simulink model "geared_motor_load_fixed"  (R2023b)
settings: Solver=VariableStepAuto  StartTime=0.0  StopTime=1  RelTol=1e-3
values from neighbouring files (symbols this model uses):
  angle_ref = Angle_reference_values(i)    [homework_three.m]
  B_load = 0    [homework_three.m]
  Beq = Jeq / 0.00376    (= 0.00264630474582)    [homework_three.m]
  gain = gear_ratio    (= 0.0123456790123)    [homework_three.m]
  gear_alpha = 0.72    [homework_three.m]
  gear_ratio = 1/81    (= 0.0123456790123)    [homework_three.m]
  J_load = 0    [homework_three.m]
  Jeq = Jm + (1 / gear_alpha) * gear_ratio * gear_ratio * Jg    (= 9.9501058443e-06)    [homework_three.m]
  Ka_c = 1 / Kp_c    (= 2.41883946985)    [homework_three.m]
  Ka_v = 1/Kp_v    (= 289.1342348)    [homework_three.m]
  Kd_p = wcp/wcv    (= 0.1)    [homework_three.m]
  Ke = 0.0683    [homework_three.m]
  Ki_c = Ra * wcc    (= 1105.808)    [homework_three.m]
  Ki_v = (Beq+(B_load*0.00021))*wcv*81/Kt    (= 197.183799438)    [homework_three.m]
  Kp_c = La * wcc    (= 0.4134214)    [homework_three.m]
  Kp_p = wcp    (= 6.283)    [homework_three.m]
  Kp_v = (Jeq+(J_load*0.00021))*wcv*81*Kt    (= 0.00345860116044)    [homework_three.m]
  Kt = 0.0683    [homework_three.m]
  La = 0.000658    [homework_three.m]
  Ra = 1.76    [homework_three.m]
settings Model: Creator=junseo  LastModifiedBy=minjs
settings SolverCC: ZeroCrossAlgorithm=Adaptive
settings OptimizationCC: ReuseModelBlockBuffer=off
settings DebuggingCC: IgnoredZcDiagnostic=none

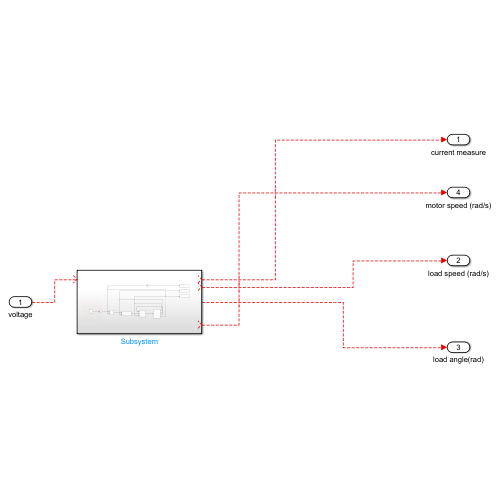
[thumbnail: Simulink's stored preview of the top-level diagram]
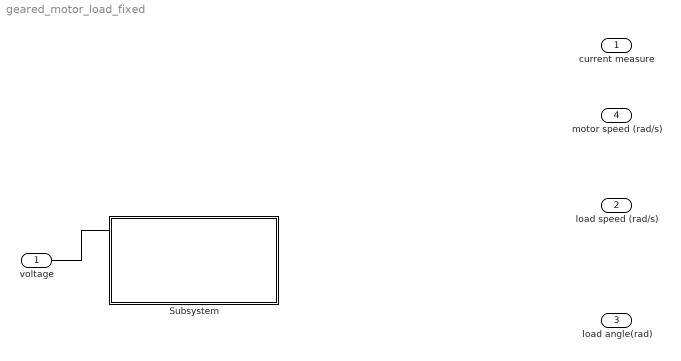
== system geared_motor_load_fixed ==
  voltage : Inport
  Subsystem : Subsystem
  current measure : Outport
  load speed (rad/s) : Outport  Port=2
  load angle(rad) : Outport  Port=3
  motor speed (rad/s) : Outport  Port=4
  wires:
  voltage/1 -> ?
  ? -> current measure/1
  ? -> load speed (rad/s)/1
  ? -> load angle(rad)/1
  ? -> motor speed (rad/s)/1

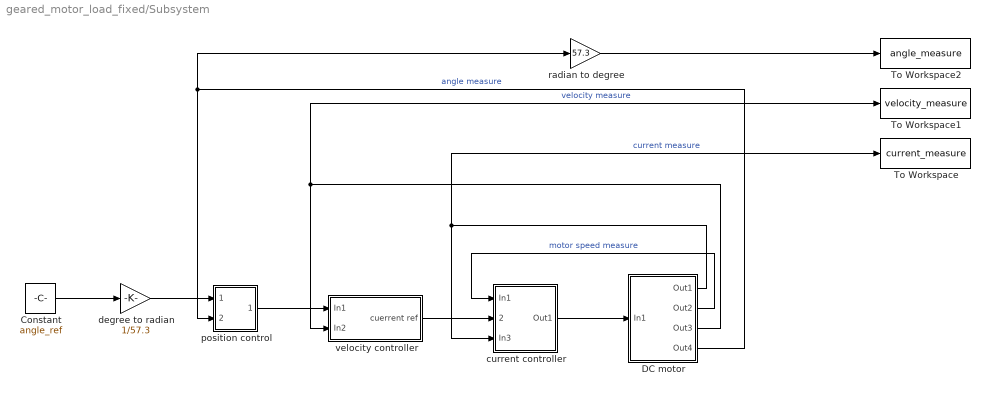
== system geared_motor_load_fixed/Subsystem ==
  Constant : Constant  Value=angle_ref
  DC motor : Subsystem
  To Workspace : ToWorkspace  VariableName=current_measure  SaveFormat=Timeseries  SampleTime=-1
  To Workspace1 : ToWorkspace  VariableName=velocity_measure  SaveFormat=Timeseries  SampleTime=-1
  To Workspace2 : ToWorkspace  VariableName=angle_measure  SaveFormat=Timeseries  SampleTime=-1
  current controller : Subsystem
  degree to radian : Gain  Gain=1/57.3
  position control : Subsystem
  radian to degree : Gain  Gain=57.3
  velocity controller : Subsystem
  wires:
  current controller/1(Out1) -> DC motor/1(In1)
  DC motor/2(Out2) -> current controller/1(In1)  "motor speed measure"
  DC motor/1(Out1) -> To Workspace/1, current controller/3(In3)  "current measure"
  position control/1(Out1) -> velocity controller/1(In1)
  DC motor/3(Out3) -> To Workspace1/1, velocity controller/2(In2)  "velocity measure"
  velocity controller/1(cuerrent ref) -> current controller/2(cuerrent ref)
  Constant/1 -> degree to radian/1
  DC motor/4(Out4) -> radian to degree/1, position control/2(In2)  "angle measure"
  radian to degree/1 -> To Workspace2/1
  degree to radian/1 -> position control/1(In1)

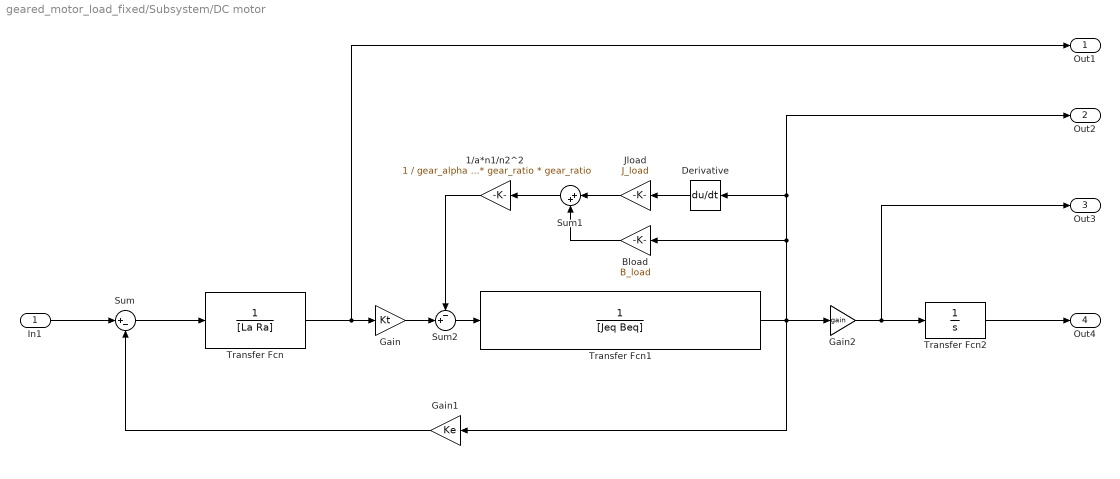
== system geared_motor_load_fixed/Subsystem/DC motor ==
  In1 : Inport
  1/a*n1/n2^2 : Gain  Gain=1 / gear_alpha * gear_ratio * gear_ratio
  Bload : Gain  Gain=B_load
  Derivative : Derivative
  Gain : Gain  Gain=Kt
  Gain1 : Gain  Gain=Ke
  Gain2 : Gain  Gain=gain
  Jload : Gain  Gain=J_load
  Sum : Sum  Inputs=|+-
  Sum1 : Sum  Inputs=|++
  Sum2 : Sum  Inputs=-+|
  Transfer Fcn : TransferFcn  Denominator=[La Ra]
  Transfer Fcn1 : TransferFcn  Denominator=[Jeq Beq]
  Transfer Fcn2 : TransferFcn  Denominator=[1 0]
  Out1 : Outport
  Out2 : Outport  Port=2
  Out3 : Outport  Port=3
  Out4 : Outport  Port=4
  wires:
  Jload/1 -> Sum1/1
  Gain1/1 -> Sum/2
  Bload/1 -> Sum1/2
  Sum2/1 -> Transfer Fcn1/1
  Gain2/1 -> Out3/1, Transfer Fcn2/1
  Derivative/1 -> Jload/1
  Transfer Fcn1/1 -> Gain1/1, Gain2/1, Bload/1, Out2/1, Derivative/1
  Transfer Fcn/1 -> Out1/1, Gain/1
  Sum1/1 -> 1/a*n1/n2^2/1
  1/a*n1/n2^2/1 -> Sum2/1
  Gain/1 -> Sum2/2
  Sum/1 -> Transfer Fcn/1
  Transfer Fcn2/1 -> Out4/1
  In1/1 -> Sum/1

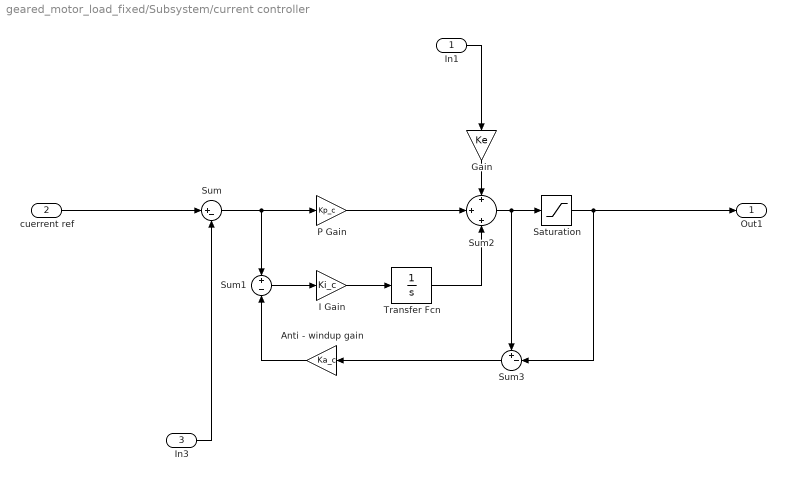
== system geared_motor_load_fixed/Subsystem/current controller ==
  In1 : Inport
  cuerrent ref : Inport  Port=2
  In3 : Inport  Port=3
  Anti - windup gain : Gain  Gain=Ka_c
  Gain : Gain  Gain=Ke
  I Gain : Gain  Gain=Ki_c
  P Gain : Gain  Gain=Kp_c
  Saturation : Saturate  UpperLimit=48  LowerLimit=-48
  Sum : Sum  Inputs=|+-
  Sum1 : Sum  Inputs=+|-
  Sum2 : Sum  Inputs=+|+|+
  Sum3 : Sum  Inputs=+-|
  Transfer Fcn : TransferFcn  Denominator=[1 0]
  Out1 : Outport
  wires:
  cuerrent ref/1 -> Sum/1
  I Gain/1 -> Transfer Fcn/1
  Transfer Fcn/1 -> Sum2/3
  Sum1/1 -> I Gain/1
  Sum/1 -> Sum1/1, P Gain/1
  Gain/1 -> Sum2/1
  P Gain/1 -> Sum2/2
  Saturation/1 -> Out1/1, Sum3/2
  In1/1 -> Gain/1
  Sum2/1 -> Saturation/1, Sum3/1
  Sum3/1 -> Anti - windup gain/1
  Anti - windup gain/1 -> Sum1/2
  In3/1 -> Sum/2

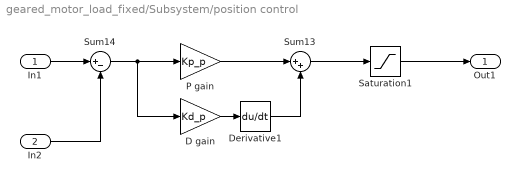
== system geared_motor_load_fixed/Subsystem/position control ==
  In1 : Inport
  In2 : Inport  Port=2
  D gain : Gain  Gain=Kd_p
  Derivative1 : Derivative
  P gain : Gain  Gain=Kp_p
  Saturation1 : Saturate  UpperLimit=643  LowerLimit=-643
  Sum13 : Sum  Inputs=|++
  Sum14 : Sum  Inputs=|+-
  Out1 : Outport
  wires:
  Saturation1/1 -> Out1/1
  P gain/1 -> Sum13/1
  Sum13/1 -> Saturation1/1
  In2/1 -> Sum14/2
  D gain/1 -> Derivative1/1
  Sum14/1 -> D gain/1, P gain/1
  Derivative1/1 -> Sum13/2
  In1/1 -> Sum14/1

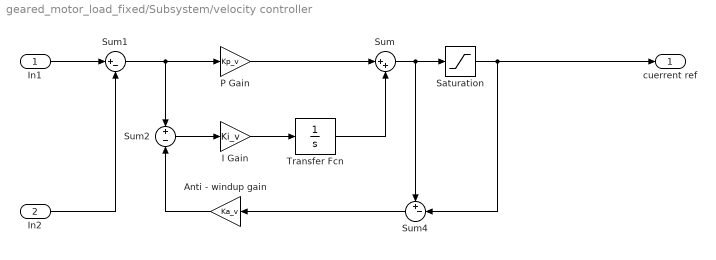
== system geared_motor_load_fixed/Subsystem/velocity controller ==
  In1 : Inport
  In2 : Inport  Port=2
  Anti - windup gain : Gain  Gain=Ka_v
  I Gain : Gain  Gain=Ki_v
  P Gain : Gain  Gain=Kp_v
  Saturation : Saturate  UpperLimit=27.3  LowerLimit=-27.3
  Sum : Sum  Inputs=|++
  Sum1 : Sum  Inputs=|+-
  Sum2 : Sum  Inputs=+|-
  Sum4 : Sum  Inputs=+-|
  Transfer Fcn : TransferFcn  Denominator=[1 0]
  cuerrent ref : Outport
  wires:
  I Gain/1 -> Transfer Fcn/1
  Sum/1 -> Saturation/1, Sum4/1
  Transfer Fcn/1 -> Sum/2
  Sum1/1 -> Sum2/1, P Gain/1
  Sum4/1 -> Anti - windup gain/1
  P Gain/1 -> Sum/1
  Saturation/1 -> cuerrent ref/1, Sum4/2
  Sum2/1 -> I Gain/1
  Anti - windup gain/1 -> Sum2/2
  In2/1 -> Sum1/2
  In1/1 -> Sum1/1
